simulink model "Combinacion"  (R2018a)
settings: Solver=FixedStepAuto  StartTime=0.0  StopTime=30  RelTol=1e-3
values from neighbouring files (symbols this model uses):
  Tm = 0.1/5    (= 0.02)    [Init.m]
libraries: simulink x2, powerlib_meascontrol x2, simulink_extras x1
settings Model: Creator=Augusto  LastModifiedBy=Augusto

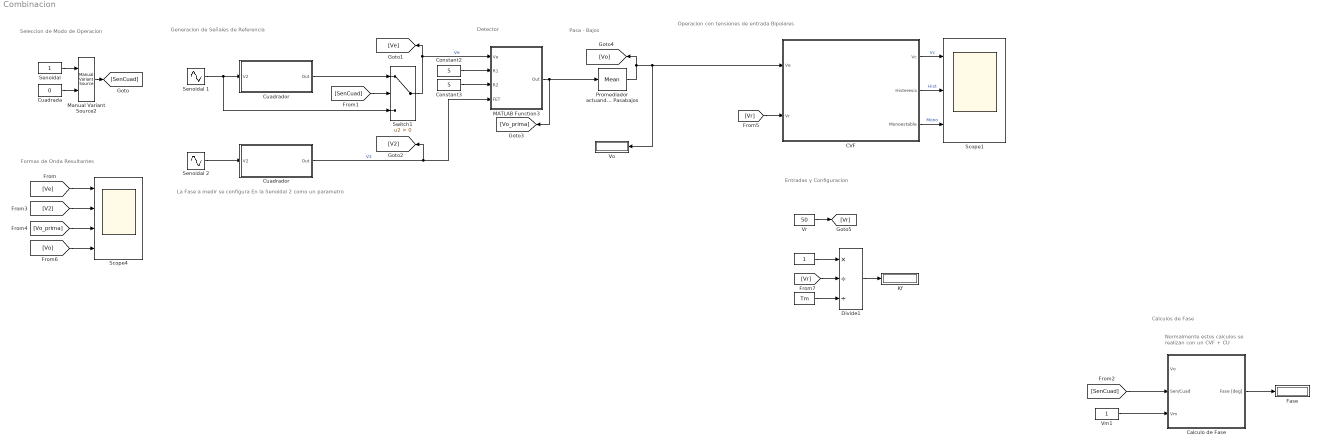
== system Combinacion ==
  note: Operacion con tensiones de entrada Bipolares
  note: Calculos de Fase
  note: Pasa - Bajos
  note: Normalmente estos calculos se
      | realizan con un CVF + CU
  note: Seleccion de Modo de Operacion
  note: Formas de Onda Resultantes
  note: Generacion de Señales de Referencia
  note: Detector
  note: La Fase a medir se configura En la Senoidal 2 como un parametro
  note: Entradas y Configuracion
  " " : Constant  Value=Tm
  "   " : Constant
  CVF : Subsystem
  Calculo de Fase : Subsystem
  Constant2 : Constant  Value=5
  Constant3 : Constant  Value=5
  Cuadrada : Constant  Value=0
  Cuadrador : MATLAB Function  TreatAsAtomicUnit=on
  "Cuadrador " : MATLAB Function  TreatAsAtomicUnit=on
  Divide1 : Product  Inputs=*//
  Fase : Display
  Kf : Display
  MATLAB Function3 : MATLAB Function  TreatAsAtomicUnit=on
  Manual Variant Source2 : simulink/Signal Routing/Manual Variant Source  NumChoices=2  OverrideUsingVariant=V_2
      settings: SourceProductName=Simulink
  Promediador actuando como Pasabajos : powerlib_meascontrol/Measurements/Mean  Freq=1  Vinit=0  Ts=0
  Scope1 : Scope  NumInputPorts=3
  Scope4 : Scope  NumInputPorts=4
  Senoidal : Constant
  Senoidal 1 : Sin  Frequency=2*pi  SampleTime=0
  Senoidal 2 : Sin  Frequency=2*pi  Phase=(pi/180)*180  SampleTime=0
  Switch1 : Switch  Criteria=u2 > Threshold
  Vm1 : Constant
  Vo : Display
  Vr : Constant  Value=50
  wires:
  CVF/2(Histeresis) -> Scope1/2  "Hist"
  CVF/1(Vc) -> Scope1/1  "Vc"
  CVF/3(Monoestable) -> Scope1/3  "Mono"
  [Vr] -> CVF/2(Vr)
  Promediador actuando como Pasabajos/1 -> CVF/1(Ve), Vo/1, [Vo]
  [SenCuad] -> Calculo de Fase/2(Sen/Cuad)
  Switch1/1 -> [Ve], MATLAB Function3/1(Ve)  "Ve"
  MATLAB Function3/1(Out) -> [Vo_prima], Promediador actuando como Pasabajos/1
  [Ve] -> Scope4/1
  [Vo] -> Scope4/4
  Constant3/1 -> MATLAB Function3/3(R2)
  [V2] -> Scope4/2
  [Vo_prima] -> Scope4/3
  Senoidal/1 -> Manual Variant Source2/1
  Senoidal 1/1 -> "Cuadrador "/1(V2), Switch1/3
  Calculo de Fase/1(Fase [deg]) -> Fase/1
  Senoidal 2/1 -> Cuadrador/1(V2)
  Constant2/1 -> MATLAB Function3/2(R1)
  Manual Variant Source2/1 -> [SenCuad]
  Cuadrada/1 -> Manual Variant Source2/2
  [SenCuad] -> Switch1/2
  Cuadrador/1(Out) -> [V2], MATLAB Function3/4(FET)  "V2"
  Vm1/1 -> Calculo de Fase/3(Vm)
  "Cuadrador "/1(Out) -> Switch1/1
  Vr/1 -> [Vr]
  Divide1/1 -> Kf/1
  [Vr] -> Divide1/2
  " "/1 -> Divide1/3
  "   "/1 -> Divide1/1

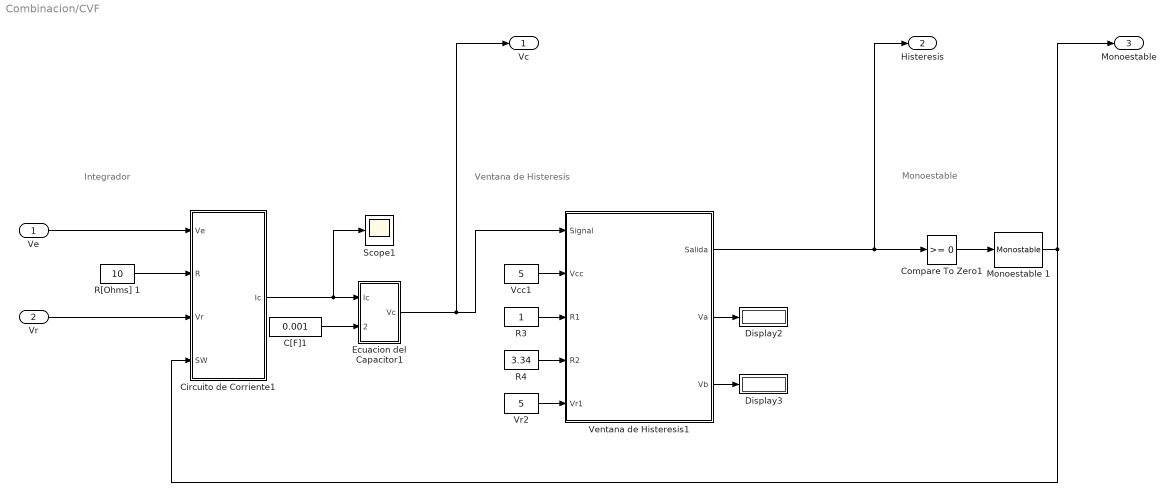
== system Combinacion/CVF ==
  note: Ventana de Histeresis
  note: Monoestable
  note: Integrador
  Ve : Inport
  Vr : Inport  Port=2
  C[F]1 : Constant  Value=0.001
  Circuito de Corriente1 : Subsystem
  Compare To Zero1 : simulink/Logic and Bit Operations/Compare To Zero  relop=>=  OutDataTypeStr=boolean
  Display2 : Display
  Display3 : Display
  Ecuacion del Capacitor1 : Subsystem
  Monoestable 1 : powerlib_meascontrol/Logic/Monostable  EdgeDetect=Falling  PulseDuration=Tm  ic=1  Ts=0
      settings: SourceProductName=Simscape Power Systems  SourceProductBaseCode=PS
  R3 : Constant
  R4 : Constant  Value=3.34
  R[Ohms] 1 : Constant  Value=10
  Scope1 : Scope
  Vcc1 : Constant  Value=5
  Ventana de Histeresis1 : MATLAB Function  TreatAsAtomicUnit=on
  Vr2 : Constant  Value=5
  Vc : Outport
  Histeresis : Outport  Port=2
  Monoestable : Outport  Port=3
  wires:
  Vcc1/1 -> Ventana de Histeresis1/2(Vcc)
  Ventana de Histeresis1/3(Vb) -> Display3/1
  Ventana de Histeresis1/2(Va) -> Display2/1
  Ventana de Histeresis1/1(Salida) -> Histeresis/1, Compare To Zero1/1
  R[Ohms] 1/1 -> Circuito de Corriente1/2(R)
  Ecuacion del Capacitor1/1(Vc) -> Vc/1, Ventana de Histeresis1/1(Signal)
  Vr2/1 -> Ventana de Histeresis1/5(Vr1)
  Compare To Zero1/1 -> Monoestable 1/1
  Circuito de Corriente1/1(Ic) -> Scope1/1, Ecuacion del Capacitor1/1(Ic)
  R3/1 -> Ventana de Histeresis1/3(R1)
  C[F]1/1 -> Ecuacion del Capacitor1/2(Cap)
  R4/1 -> Ventana de Histeresis1/4(R2)
  Vr/1 -> Circuito de Corriente1/3(Vr)
  Monoestable 1/1 -> Monoestable/1, Circuito de Corriente1/4(SW)
  Ve/1 -> Circuito de Corriente1/1(Ve)

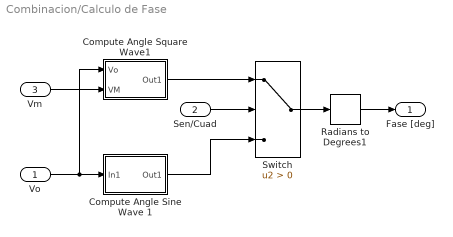
== system Combinacion/Calculo de Fase ==
  Vo : Inport
  Sen/Cuad : Inport  Port=2
  Vm : Inport  Port=3
  Compute Angle Sine Wave 1 : Subsystem
  Compute Angle Square Wave1 : Subsystem
  Radians to Degrees1 : simulink_extras/Transformations/Radians to Degrees
  Switch : Switch  Criteria=u2 > Threshold
  Fase [deg] : Outport
  wires:
  Vm/1 -> Compute Angle Square Wave1/2(VM)
  Switch/1 -> Radians to Degrees1/1
  Radians to Degrees1/1 -> Fase [deg]/1
  Vo/1 -> Compute Angle Square Wave1/1("Vo "), Compute Angle Sine Wave 1/1(In1)
  Sen/Cuad/1 -> Switch/2
  Compute Angle Sine Wave 1/1(Out1) -> Switch/3
  Compute Angle Square Wave1/1(Out1) -> Switch/1

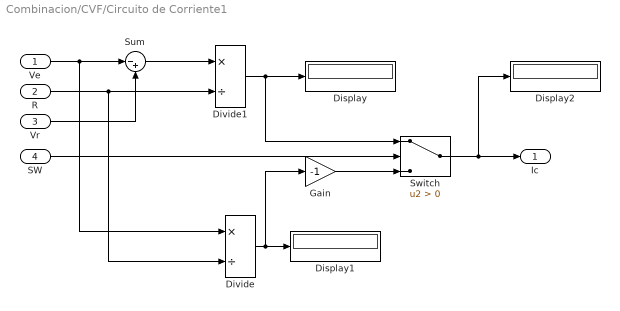
== system Combinacion/CVF/Circuito de Corriente1 ==
  Ve : Inport
  R : Inport  Port=2
  Vr : Inport  Port=3
  SW : Inport  Port=4
  Display : Display
  Display1 : Display
  Display2 : Display
  Divide : Product  Inputs=*/
  Divide1 : Product  Inputs=*/
  Gain : Gain  Gain=-1
  Sum : Sum  Inputs=|-+
  Switch : Switch  Criteria=u2 > Threshold
  Ic : Outport
  wires:
  Ve/1 -> Divide/1, Sum/1
  SW/1 -> Switch/2
  Sum/1 -> Divide1/1
  Divide/1 -> Display1/1, Gain/1
  Divide1/1 -> Display/1, Switch/1
  Vr/1 -> Sum/2
  R/1 -> Divide/2, Divide1/2
  Switch/1 -> Display2/1, Ic/1
  Gain/1 -> Switch/3

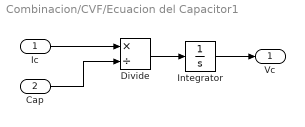
== system Combinacion/CVF/Ecuacion del Capacitor1 ==
  Ic : Inport
  Cap : Inport  Port=2
  Divide : Product  Inputs=*/
  Integrator : Integrator
  Vc : Outport
  wires:
  Ic/1 -> Divide/1
  Integrator/1 -> Vc/1
  Divide/1 -> Integrator/1
  Cap/1 -> Divide/2

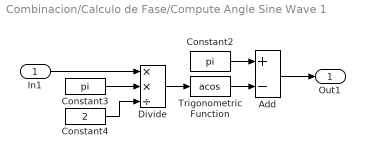
== system Combinacion/Calculo de Fase/Compute Angle Sine Wave 1 ==
  In1 : Inport
  Add : Sum  Inputs=+-
  Constant2 : Constant  Value=pi
  Constant3 : Constant  Value=pi
  Constant4 : Constant  Value=2
  Divide : Product  Inputs=**/
  Trigonometric Function : Trigonometry  Operator=acos
  Out1 : Outport
  wires:
  Constant2/1 -> Add/1
  In1/1 -> Divide/1
  Constant3/1 -> Divide/2
  Divide/1 -> Trigonometric Function/1
  Constant4/1 -> Divide/3
  Trigonometric Function/1 -> Add/2
  Add/1 -> Out1/1

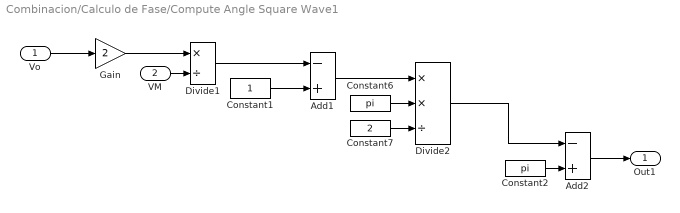
== system Combinacion/Calculo de Fase/Compute Angle Square Wave1 ==
  "Vo " : Inport
  VM : Inport  Port=2
  Add1 : Sum  Inputs=-+
  Add2 : Sum  Inputs=-+
  Constant1 : Constant
  Constant2 : Constant  Value=pi
  Constant6 : Constant  Value=pi
  Constant7 : Constant  Value=2
  Divide1 : Product  Inputs=*/
  Divide2 : Product  Inputs=**/
  Gain : Gain  Gain=2
  Out1 : Outport
  wires:
  "Vo "/1 -> Gain/1
  VM/1 -> Divide1/2
  Divide1/1 -> Add1/1
  Constant1/1 -> Add1/2
  Constant7/1 -> Divide2/3
  Constant6/1 -> Divide2/2
  Add1/1 -> Divide2/1
  Gain/1 -> Divide1/1
  Divide2/1 -> Add2/1
  Add2/1 -> Out1/1
  Constant2/1 -> Add2/2

== matlab function Combinacion/CVF/Ventana de Histeresis1 ==
  settings: updateMethod=DISCRETE
  data: Signal input; Salida output; Vcc input; R1 input; R2 input; Vr1 input; Va output; Vb output
function [Salida,Va,Vb]= fcn(Signal,Vcc,R1,R2,Vr1)
     
    persistent u 
    if isempty(u)
        u=Vcc;
        Va = 0;
        Vb = 0;
    
    else
        epsilon = Vcc*(R1/R2);
        VR1 = -Vr1*(R1+R2)/R2;
        Va = VR1 - epsilon;
        Vb = VR1 + epsilon;
        if(Signal<=Va) 
            u = -Vcc;
        end
        if(Signal>=Vb)
            u = Vcc;
        end
    end
    
    Salida = u;

== matlab function Combinacion/MATLAB Function3 ==
  data: Ve input; Out output; R1 input; R2 input; FET input
function Out = Detector(Ve,R1,R2,FET)
    if FET
        Out = (-R2/R1)*Ve;
    else
        Out = Ve;
    end

== matlab function Combinacion/Cuadrador ==
  data: V2 input; Out output
function Out = CuadradorDeReferencia(V2)
    if V2 >=0
        Out = 1;
    else
        Out = 0;
    end

== matlab function Combinacion/Cuadrador  ==
  data: V2 input; Out output
function Out = CuadradorDeReferencia(V2)
    if V2 >=0
        Out = 1;
    else
        Out = 0;
    end
